simulink model "controller"  (R2022b)
settings: Solver=FixedStepAuto  StartTime=0.0  StopTime=40.0  FixedStep=0.01  RelTol=1e-3
model workspace (MAT data in the model file):
  Ki = Simulink.Parameter
  Ki.Value = 1
  Ki.DataType = 'auto'
  Ki.Complexity = 'real'
  Ki.Dimensions = [1 1]
  Kp = Simulink.Parameter
  Kp.Value = 10
  Kp.DataType = 'auto'
  Kp.Complexity = 'real'
  Kp.Dimensions = [1 1]
  Ts = Simulink.Parameter
  Ts.Value = 0.01
  Ts.DataType = 'auto'
  Ts.Complexity = 'real'
  Ts.Dimensions = [1 1]
  k = Simulink.Parameter
  k.Value = 1
  k.DataType = 'auto'
  k.Complexity = 'real'
  k.Dimensions = [1 1]
settings Model: Creator=eppa1  LastModifiedBy=eppa1

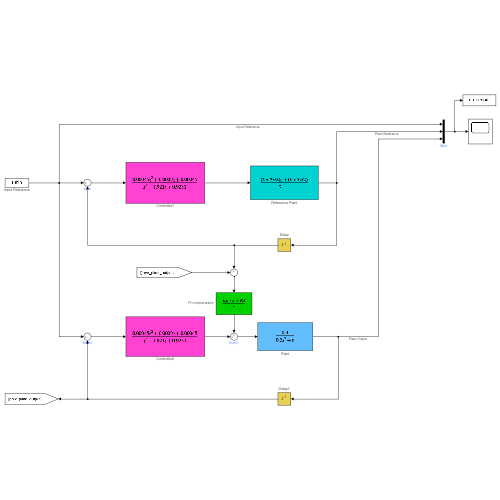
[thumbnail: Simulink's stored preview of the top-level diagram]
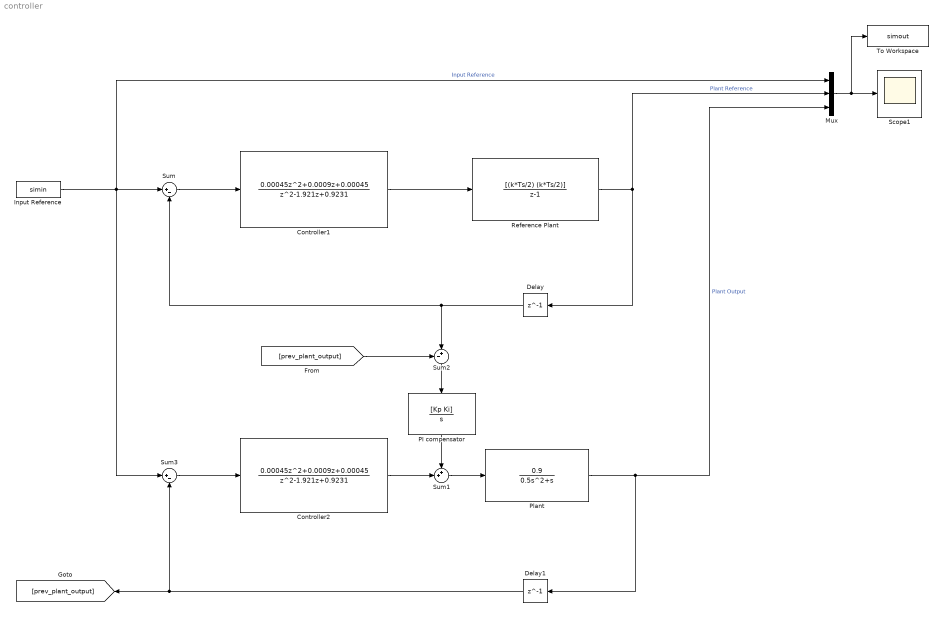
== system controller ==
  Controller1 : DiscreteTransferFcn  Numerator=[0.00045 0.0009 0.00045]  Denominator=[1 -1.921 0.9231]
  Controller2 : DiscreteTransferFcn  Numerator=[0.00045 0.0009 0.00045]  Denominator=[1 -1.921 0.9231]
  Delay : Delay  DelayLength=1
  Delay1 : Delay  DelayLength=1
  Input Reference : FromWorkspace  VariableName=simin
  Mux : Mux  Inputs=3
  PI compensator : TransferFcn  Numerator=[Kp Ki]  Denominator=[1 0]
  Plant : TransferFcn  Numerator=[0.9]  Denominator=[0.5 1 0]
  Reference Plant : DiscreteTransferFcn  Numerator=[(k*Ts/2) (k*Ts/2)]  Denominator=[1 -1]
  Scope1 : Scope
  Sum : Sum  Inputs=|+-
  Sum1 : Sum  Inputs=++|
  Sum2 : Sum  Inputs=-+|
  Sum3 : Sum  Inputs=|+-
  To Workspace : ToWorkspace  VariableName=simout  SaveFormat=Timeseries  SampleTime=-1
  wires:
  Sum/1 -> Controller1/1
  Controller1/1 -> Reference Plant/1
  Reference Plant/1 -> Mux/2, Delay/1  "Plant Reference"
  Delay/1 -> Sum2/2, Sum/2
  Input Reference/1 -> Mux/1, Sum/1, Sum3/1  "Input Reference"
  Controller2/1 -> Sum1/2
  Sum1/1 -> Plant/1
  PI compensator/1 -> Sum1/1
  Sum2/1 -> PI compensator/1
  Sum3/1 -> Controller2/1
  Plant/1 -> Mux/3, Delay1/1  "Plant Output"
  Delay1/1 -> [prev_plant_output], Sum3/2
  [prev_plant_output] -> Sum2/1
  Mux/1 -> Scope1/1, To Workspace/1
